simulink model "KiBaM2"  (R2017b)
settings: Solver=VariableStepAuto  StartTime=0.0  StopTime=200  RelTol=1e-3
settings Model: Creator=barbot  LastModifiedBy=barbot

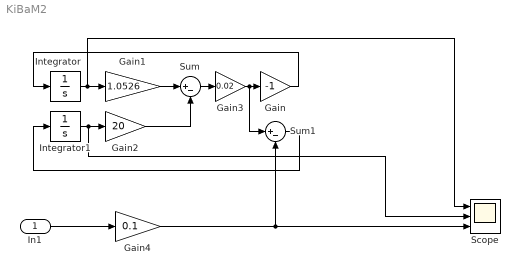
== system KiBaM2 ==
  In1 : Inport
  Gain : Gain  Gain=-1
  Gain1 : Gain  Gain=1.0526
  Gain2 : Gain  Gain=20
  Gain3 : Gain  Gain=0.02
  Gain4 : Gain  Gain=0.1
  Integrator : Integrator  InitialCondition=9.5
  Integrator1 : Integrator  InitialCondition=0.5
  Scope : Scope  NumInputPorts=3
  Sum : Sum  Inputs=|+-
  Sum1 : Sum  Inputs=|+-
  wires:
  Sum/1 -> Gain3/1
  Gain1/1 -> Sum/1
  Gain2/1 -> Sum/2
  Gain/1 -> Integrator/1
  Gain3/1 -> Sum1/1, Gain/1
  In1/1 -> Gain4/1
  Sum1/1 -> Integrator1/1
  Gain4/1 -> Sum1/2, Scope/3
  Integrator/1 -> Scope/1, Gain1/1
  Integrator1/1 -> Scope/2, Gain2/1
